simulink model "a2ae2"  (R2021a)
settings: Solver=FixedStepAuto  StartTime=0.0  StopTime=40000  RelTol=1e-3
settings Model: EnablePacing=on  Creator=Ans Shahzad  LastModifiedBy=Ans Shahzad
settings ConfigComp: DVTestSuiteOptimization=Auto  DVDetectOutOfBounds=on

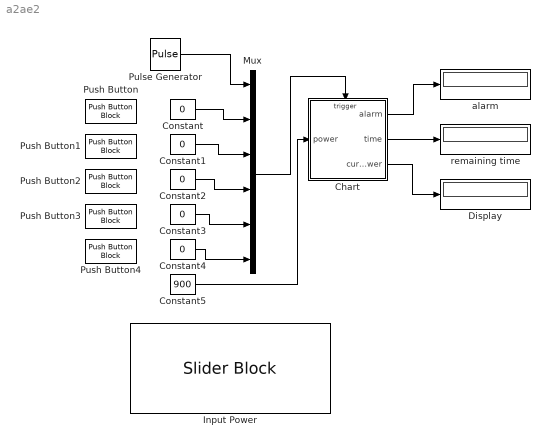
== system a2ae2 ==
  Chart : Stateflow chart  TreatAsAtomicUnit=on
  Constant{,1..4} (5 alike) : Constant  Value=0
  Constant5 : Constant  Value=900
  Display : Display
  Input Power : SliderBlock  ScaleMax=900  TickInterval=100
  Mux : Mux  Inputs=6
  Pulse Generator : DiscretePulseGenerator  PulseType=Time based  Period=1  PulseWidth=10
  Push Button : PushButtonBlock  ButtonText=Up
  Push Button1 : PushButtonBlock  ButtonText=Down
  Push Button2 : PushButtonBlock  ButtonText=Start
  Push Button3 : PushButtonBlock  ButtonText=Stop
  Push Button4 : PushButtonBlock  ButtonText=Door Open
  alarm : Display
  remaining time : Display
  wires:
  Pulse Generator/1 -> Mux/1
  Constant/1 -> Mux/2
  Constant1/1 -> Mux/3
  Constant2/1 -> Mux/4
  Constant3/1 -> Mux/5
  Chart/2(time) -> remaining time/1
  Constant4/1 -> Mux/6
  Mux/1 -> Chart/Trigger
  Chart/1(alarm) -> alarm/1
  Constant5/1 -> Chart/1(power)
  Chart/3(cur_power) -> Display/1

== stateflow chart a2ae2/Chart ==
  state Microwave
    en: alarm = false; time = 0; time = 0; cur_power = 0;
    state Normal [parallel]
      settings: executionOrder=1
      state Idling
        on Up: time = mod(time + 1, 1000);
        on Down: time = mod(time - 1, 1000);
        on TIC: cur_power = power;
      state Cooking
        on TIC: time = time  -1;
        on Up: time = mod(time + 1, 1000);
        on Down: time = mod(time- 1, 1000);
        on TIC: cur_power = power;
      state Stop
        on Stop: time = 0; time = 0; cur_power = 0;
      (default) -> Idling
      Idling -> Cooking [order 2] : Start
      Cooking -> Idling [order 1] : Door_open
      Idling -> Stop [order 1] : after(300,sec)[time > 0]{time = 0;}
      Cooking -> Stop [order 2] : Stop
      Cooking -> Stop [order 3] : [time == 0]{alarm = true; cur_power = 0;}
    state Alarm [parallel]
      settings: executionOrder=2
      state Sound
        state on
          en: alarm = true;
        state off
          en: alarm = false;
        (default) -> on
        off -> on : [after(1,sec)]
        on -> off : [after(1,sec)]
      state Idle
      (default) -> Idle
      Idle -> Sound : [alarm == true]
      Sound -> Idle : [after(5, sec)]{alarm = false}
  (default) -> Microwave
  data: alarm output boolean; time output; power input; cur_power output
  events: TIC input RISING_EDGE_EVENT; Up input RISING_EDGE_EVENT; Down input RISING_EDGE_EVENT; Start input RISING_EDGE_EVENT; Stop input RISING_EDGE_EVENT; Door_open input RISING_EDGE_EVENT
